simulink model "probe"  (R2021a)
settings: Solver=VariableStepAuto  StartTime=0.0  StopTime=100  RelTol=1e-3
values from neighbouring files (symbols this model uses):
  V1 = 1    [test.m]
  V2 = V2-0.1    (= 2.77555756156e-17)    [test.m]
settings Model: Creator=telecom  LastModifiedBy=telecom
settings DataIOCC: ReturnWorkspaceOutputs=off

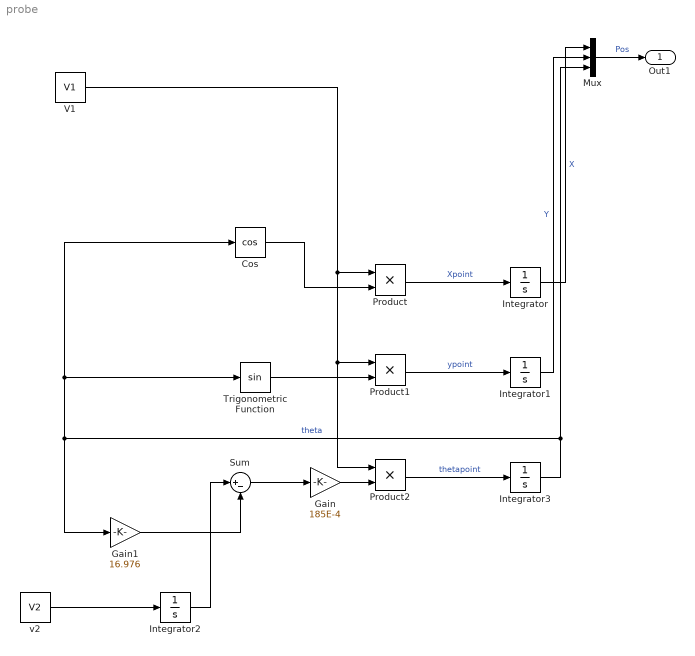
== system probe ==
  Cos : Trigonometry  Operator=cos
  Gain : Gain  Gain=185E-4
  Gain1 : Gain  Gain=16.976
  Integrator{,1..3} (4 alike) : Integrator
  Mux : Mux  Inputs=3
  Product : Product
  Product1 : Product
  Product2 : Product
  Sum : Sum  Inputs=|+-
  Trigonometric Function : Trigonometry
  V1 : Constant  Value=V1
  v2 : Constant  Value=V2
  Out1 : Outport
  wires:
  V1/1 -> Product2/1, Product1/1, Product/1
  Cos/1 -> Product/2
  Product/1 -> Integrator/1  "Xpoint"
  Trigonometric Function/1 -> Product1/2
  Product1/1 -> Integrator1/1  "ypoint"
  Gain/1 -> Product2/2
  Sum/1 -> Gain/1
  Gain1/1 -> Sum/2
  v2/1 -> Integrator2/1
  Integrator2/1 -> Sum/1
  Product2/1 -> Integrator3/1  "thetapoint"
  Integrator3/1 -> Mux/3, Trigonometric Function/1, Cos/1, Gain1/1  "theta"
  Integrator/1 -> Mux/1  "X"
  Integrator1/1 -> Mux/2  "Y"
  Mux/1 -> Out1/1  "Pos"
